simulink model "chenEx3p3p3_original"  (R2014a)
settings: Solver=ode45  StartTime=0.0  StopTime=10.0  RelTol=1e-3
values from neighbouring files (symbols this model uses):
  A = [-3.6         0       0   0 ... (first row only)    [chenEx3p3p3.m]    (also in chenEx3p3p3V3.m)
  B = [ 1 0 0 ... (first row only)    [chenEx3p3p3.m]    (also in chenEx3p3p3V3.m)
  C = [1    0   0   0 ... (first row only)    [chenEx3p3p3.m]    (also in chenEx3p3p3V3.m)
  C1 = C    [chenEx3p3p3.m]    (also in chenEx3p3p3V3.m)
  C2 = C    [chenEx3p3p3V3.m]
  C3 = C    [chenEx3p3p3V3.m]
  E = [1;20.758;0;0]    [chenEx3p3p3.m]    (also in chenEx3p3p3V3.m)
  F = A1-k1*C    [chenEx3p3p3.m]    (also in chenEx3p3p3V3.m)
  F1 = T1*A-k1*C    [chenEx3p3p3.m]    (also in chenEx3p3p3V3.m)
  H = E*inv((C*E)'*(C*E))*(C*E)'    [chenEx3p3p3.m]    (also in chenEx3p3p3V3.m)
  H1 = E1*inv((C*E1)'*(C*E1))*(C*E1)'    [chenEx3p3p3.m]    (also in chenEx3p3p3V3.m)
  H2 = E2*inv((C*E2)'*(C*E2))*(C*E2)'    [chenEx3p3p3.m]    (also in chenEx3p3p3V3.m)
  H3 = E3*inv((C*E3)'*(C*E3))*(C*E3)'    [chenEx3p3p3V3.m]
  k = k1 + F*H    [chenEx3p3p3.m]    (also in chenEx3p3p3V3.m)
  K1 = k1+F1*H1    [chenEx3p3p3.m]    (also in chenEx3p3p3V3.m)
  K2 = k2+F2*H2    [chenEx3p3p3.m]    (also in chenEx3p3p3V3.m)
  K3 = k3+F3*H3    [chenEx3p3p3V3.m]
  T = eye(4)-H*C    [chenEx3p3p3.m]    (also in chenEx3p3p3V3.m)
  T1 = eye(4) - H1*C    [chenEx3p3p3.m]    (also in chenEx3p3p3V3.m)
  T2 = eye(4) - H2*C    [chenEx3p3p3.m]    (also in chenEx3p3p3V3.m)
  T3 = eye(4) - H3*C    [chenEx3p3p3V3.m]
undefined symbols (not defined in the file or in its folder): C4, F4, H4, K, K4, T4
settings Model: Creator=sqn4594  LastModifiedBy=sqn4594
settings DataIOCC: SignalLoggingSaveFormat=ModelDataLogs
settings OptimizationCC: InitFltsAndDblsToZero=on
settings DebuggingCC: SaveWithParameterizedLinksMsg=none  UnderspecifiedInitializationDetection=Classic  SignalResolutionControl=TryResolveAllWithWarning  MultiTaskDSMMsg=warning  MultiTaskCondExecSysMsg=none
settings RTWCC: IncludeERTFirstTime=on
settings GRTTargetCC: TargetFcnLib=ansi_tfl_tmw.mat  CombineOutputUpdateFcns=off  GRTInterface=on

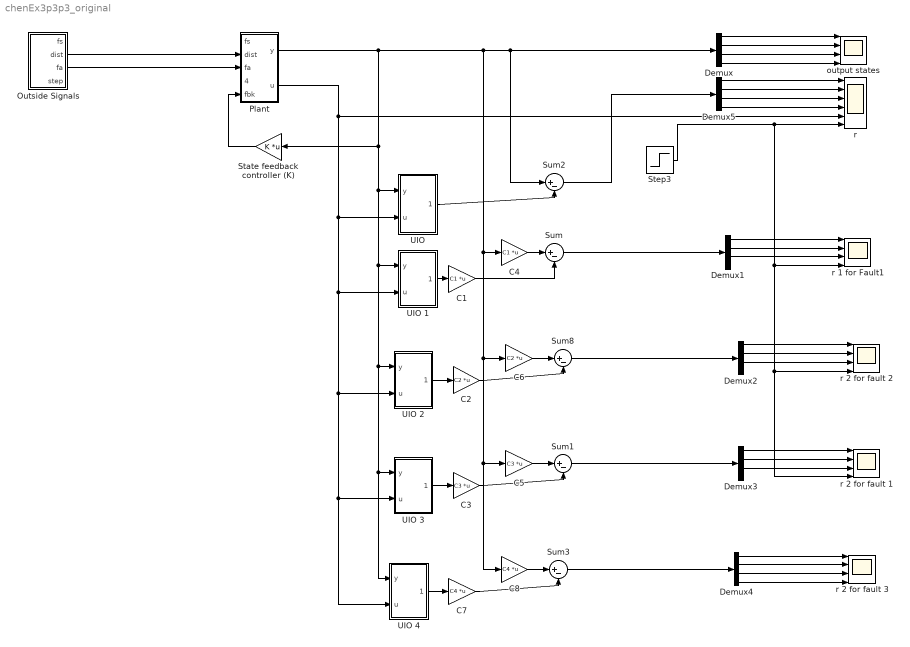
== system chenEx3p3p3_original ==
  C1 : Gain  Gain=C1  Multiplication=Matrix(K*u)
  C2 : Gain  Gain=C2  Multiplication=Matrix(K*u)
  C3 : Gain  Gain=C3  Multiplication=Matrix(K*u)
  C4 : Gain  Gain=C1  Multiplication=Matrix(K*u)
  C5 : Gain  Gain=C3  Multiplication=Matrix(K*u)
  C6 : Gain  Gain=C2  Multiplication=Matrix(K*u)
  C7 : Gain  Gain=C4  Multiplication=Matrix(K*u)
  C8 : Gain  Gain=C4  Multiplication=Matrix(K*u)
  Demux{,1..5} (6 alike) : Demux
  Outside Signals : Subsystem
  Plant : Subsystem
  State feedback controller (K) : Gain  Gain=K  Multiplication=Matrix(K*u)
  Step3 : Step  Time=7  SampleTime=0
  Sum{,1..3,8} (5 alike) : Sum  Inputs=|+-
  UIO : Subsystem
  UIO 1 : Subsystem
  UIO 2 : Subsystem
  UIO 3 : Subsystem
  UIO 4 : Subsystem
  output states : Scope  NumInputPorts=4
      settings: TimeRange=10  YMin=-5~-5~-5~-5  YMax=5~5~5~5
  r : Scope  NumInputPorts=6
      settings: YMin=-5~-5~-5~-5~-5~-5  YMax=5~5~5~5~5~5  SaveName=ScopeData5
  r 1 for Fault1 : Scope  NumInputPorts=4
      settings: YMin=-1e-020~-5~-5~-5  YMax=1e-020~5~5~5
  r 2 for fault 1 : Scope  NumInputPorts=4
      settings: YMin=-5~-5~-5~-5  YMax=5~5~5~5  SaveName=ScopeData3
  r 2 for fault 2 : Scope  NumInputPorts=4
      settings: YMin=-5~-5~-5~-5  YMax=5~5~5~5  SaveName=ScopeData2
  r 2 for fault 3 : Scope  NumInputPorts=4
      settings: YMin=-5~-5~-5~-5  YMax=5~5~5~5  SaveName=ScopeData4
  wires:
  Plant/1(y) -> State feedback controller (K)/1, UIO/1(y), UIO 1/1(y), UIO 2/1(y), UIO 3/1(y), UIO 4/1(y), Demux/1, Sum2/1, C4/1, C6/1, C5/1, C8/1
  Demux/2 -> output states/2
  Demux/3 -> output states/3
  Demux/4 -> output states/4
  Demux1/1 -> r 1 for Fault1/1
  State feedback controller (K)/1 -> Plant/5(fbk)
  Plant/2(u) -> UIO/2(u), UIO 1/2(u), UIO 2/2(u), UIO 3/2(u), UIO 4/2(u), r/5
  Step3/1 -> r/6, r 1 for Fault1/4, r 2 for fault 2/4, r 2 for fault 1/4
  UIO/1(ydot) -> Sum2/2
  Demux5/1 -> r/1
  Demux5/2 -> r/2
  Demux5/3 -> r/3
  Demux5/4 -> r/4
  Sum2/1 -> Demux5/1
  Demux/1 -> output states/1
  UIO 1/1(xdot) -> C1/1
  C1/1 -> Sum/2
  Demux1/2 -> r 1 for Fault1/2
  Demux1/3 -> r 1 for Fault1/3
  Sum/1 -> Demux1/1
  C4/1 -> Sum/1
  UIO 2/1(xdot) -> C2/1
  Demux2/1 -> r 2 for fault 2/1
  Demux2/2 -> r 2 for fault 2/2
  Demux2/3 -> r 2 for fault 2/3
  Sum8/1 -> Demux2/1
  C2/1 -> Sum8/2
  C6/1 -> Sum8/1
  UIO 3/1(xdot) -> C3/1
  Demux3/1 -> r 2 for fault 1/1
  Demux3/2 -> r 2 for fault 1/2
  Demux3/3 -> r 2 for fault 1/3
  Sum1/1 -> Demux3/1
  C3/1 -> Sum1/2
  C5/1 -> Sum1/1
  UIO 4/1(xdot) -> C7/1
  Demux4/1 -> r 2 for fault 3/1
  Demux4/2 -> r 2 for fault 3/2
  Demux4/3 -> r 2 for fault 3/3
  Sum3/1 -> Demux4/1
  C7/1 -> Sum3/2
  Demux4/4 -> r 2 for fault 3/4
  C8/1 -> Sum3/1
  Outside Signals/3(fa) -> Plant/3(fa)
  Outside Signals/2(dist) -> Plant/2(dist)

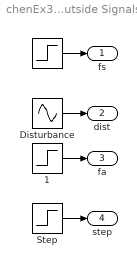
== system chenEx3p3p3_original/Outside Signals ==
  "  " : Step  Time=7  SampleTime=0
  "  1" : Step  Time=7  SampleTime=0
  Disturbance : Sin  Frequency=100  SampleTime=0
  Step : Step  Time=0  SampleTime=0
  fs : Outport
  dist : Outport  Port=2
  fa : Outport  Port=3
  "step " : Outport  Port=4
  wires:
  "  "/1 -> fs/1
  Disturbance/1 -> dist/1
  "  1"/1 -> fa/1
  Step/1 -> "step "/1

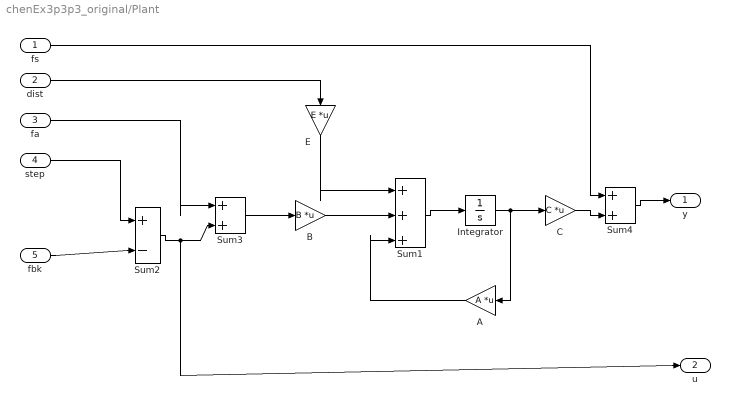
== system chenEx3p3p3_original/Plant ==
  fs : Inport
  dist : Inport  Port=2
  fa : Inport  Port=3
  step : Inport  Port=4
  fbk : Inport  Port=5
  A : Gain  Gain=A  Multiplication=Matrix(K*u)
  B : Gain  Gain=B  Multiplication=Matrix(K*u)
  C : Gain  Gain=C  Multiplication=Matrix(K*u)
  E : Gain  Gain=E  Multiplication=Matrix(K*u)
  Integrator : Integrator  InitialCondition=[.01;0;.011;.011]
  Sum1 : Sum  Inputs=|+++
  Sum2 : Sum  Inputs=|+-
  Sum3 : Sum  Inputs=|++
  Sum4 : Sum  Inputs=|++
  y : Outport
  u : Outport  Port=2
  wires:
  Sum1/1 -> Integrator/1
  step/1 -> Sum2/1
  fbk/1 -> Sum2/2
  Integrator/1 -> C/1, A/1
  Sum2/1 -> Sum3/2, u/1
  B/1 -> Sum1/2
  Sum3/1 -> B/1
  C/1 -> Sum4/2
  A/1 -> Sum1/3
  E/1 -> Sum1/1
  Sum4/1 -> y/1
  fa/1 -> Sum3/1
  dist/1 -> E/1
  fs/1 -> Sum4/1

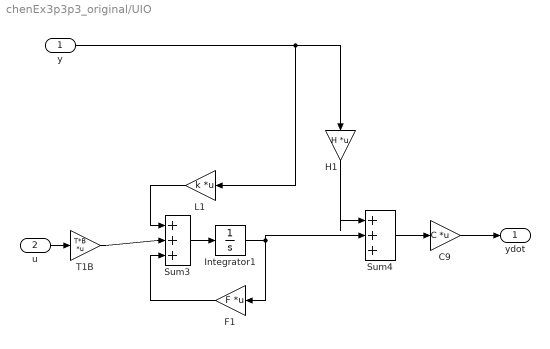
== system chenEx3p3p3_original/UIO ==
  y : Inport
  u : Inport  Port=2
  C9 : Gain  Gain=C  Multiplication=Matrix(K*u)
  F1 : Gain  Gain=F  Multiplication=Matrix(K*u)
  H1 : Gain  Gain=H  Multiplication=Matrix(K*u)
  Integrator1 : Integrator
  L1 : Gain  Gain=k  Multiplication=Matrix(K*u)
  Sum3 : Sum  Inputs=|+++
  Sum4 : Sum  Inputs=|+++
  T1B : Gain  Gain=T*B  Multiplication=Matrix(K*u)
  ydot : Outport
  wires:
  Sum3/1 -> Integrator1/1
  Integrator1/1 -> F1/1, Sum4/2
  F1/1 -> Sum3/3
  L1/1 -> Sum3/1
  T1B/1 -> Sum3/2
  H1/1 -> Sum4/1
  Sum4/1 -> C9/1
  y/1 -> L1/1, H1/1
  u/1 -> T1B/1
  C9/1 -> ydot/1

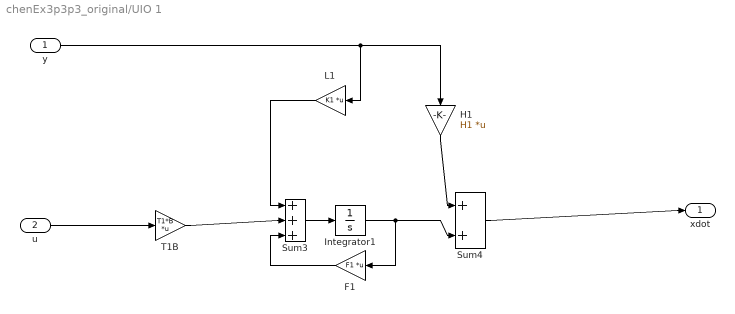
== system chenEx3p3p3_original/UIO 1 ==
  y : Inport
  u : Inport  Port=2
  F1 : Gain  Gain=F1  Multiplication=Matrix(K*u)
  H1 : Gain  Gain=H1  Multiplication=Matrix(K*u)
  Integrator1 : Integrator
  L1 : Gain  Gain=K1  Multiplication=Matrix(K*u)
  Sum3 : Sum  Inputs=|+++
  Sum4 : Sum  Inputs=|++
  T1B : Gain  Gain=T1*B  Multiplication=Matrix(K*u)
  xdot : Outport
  wires:
  Sum3/1 -> Integrator1/1
  Integrator1/1 -> Sum4/2, F1/1
  F1/1 -> Sum3/3
  L1/1 -> Sum3/1
  T1B/1 -> Sum3/2
  H1/1 -> Sum4/1
  u/1 -> T1B/1
  Sum4/1 -> xdot/1
  y/1 -> H1/1, L1/1

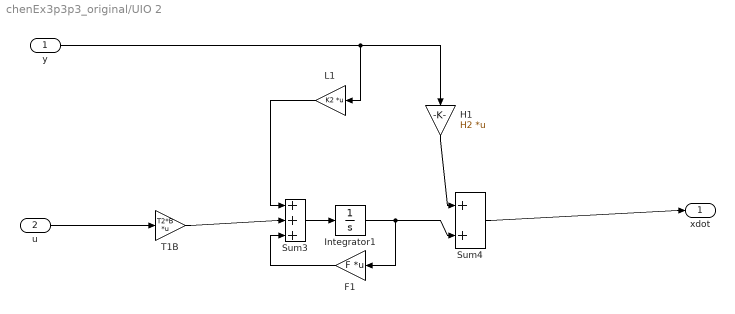
== system chenEx3p3p3_original/UIO 2 ==
  y : Inport
  u : Inport  Port=2
  F1 : Gain  Gain=F  Multiplication=Matrix(K*u)
  H1 : Gain  Gain=H2  Multiplication=Matrix(K*u)
  Integrator1 : Integrator
  L1 : Gain  Gain=K2  Multiplication=Matrix(K*u)
  Sum3 : Sum  Inputs=|+++
  Sum4 : Sum  Inputs=|++
  T1B : Gain  Gain=T2*B  Multiplication=Matrix(K*u)
  xdot : Outport
  wires:
  Sum3/1 -> Integrator1/1
  Integrator1/1 -> Sum4/2, F1/1
  F1/1 -> Sum3/3
  L1/1 -> Sum3/1
  T1B/1 -> Sum3/2
  H1/1 -> Sum4/1
  u/1 -> T1B/1
  Sum4/1 -> xdot/1
  y/1 -> H1/1, L1/1

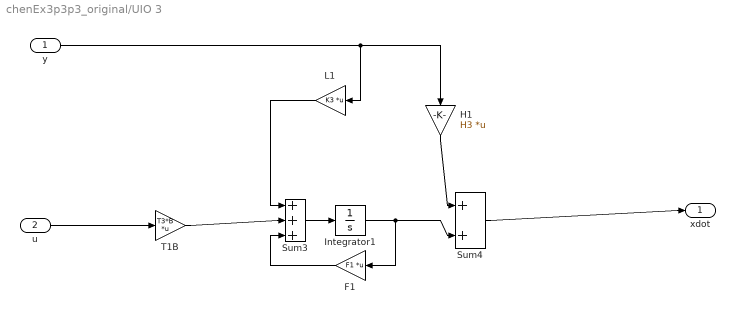
== system chenEx3p3p3_original/UIO 3 ==
  y : Inport
  u : Inport  Port=2
  F1 : Gain  Gain=F1  Multiplication=Matrix(K*u)
  H1 : Gain  Gain=H3  Multiplication=Matrix(K*u)
  Integrator1 : Integrator
  L1 : Gain  Gain=K3  Multiplication=Matrix(K*u)
  Sum3 : Sum  Inputs=|+++
  Sum4 : Sum  Inputs=|++
  T1B : Gain  Gain=T3*B  Multiplication=Matrix(K*u)
  xdot : Outport
  wires:
  Sum3/1 -> Integrator1/1
  Integrator1/1 -> Sum4/2, F1/1
  F1/1 -> Sum3/3
  L1/1 -> Sum3/1
  T1B/1 -> Sum3/2
  H1/1 -> Sum4/1
  u/1 -> T1B/1
  Sum4/1 -> xdot/1
  y/1 -> H1/1, L1/1

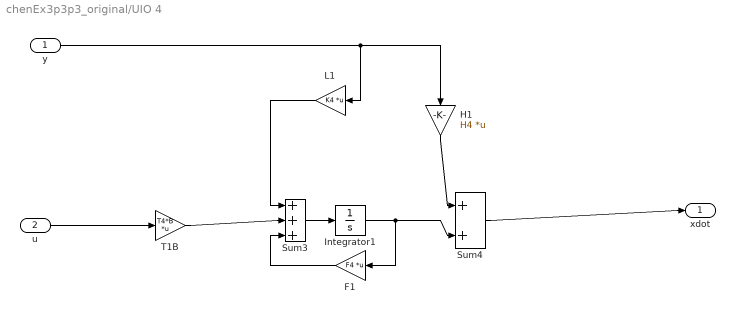
== system chenEx3p3p3_original/UIO 4 ==
  y : Inport
  u : Inport  Port=2
  F1 : Gain  Gain=F4  Multiplication=Matrix(K*u)
  H1 : Gain  Gain=H4  Multiplication=Matrix(K*u)
  Integrator1 : Integrator
  L1 : Gain  Gain=K4  Multiplication=Matrix(K*u)
  Sum3 : Sum  Inputs=|+++
  Sum4 : Sum  Inputs=|++
  T1B : Gain  Gain=T4*B  Multiplication=Matrix(K*u)
  xdot : Outport
  wires:
  Sum3/1 -> Integrator1/1
  Integrator1/1 -> Sum4/2, F1/1
  F1/1 -> Sum3/3
  L1/1 -> Sum3/1
  T1B/1 -> Sum3/2
  H1/1 -> Sum4/1
  u/1 -> T1B/1
  Sum4/1 -> xdot/1
  y/1 -> H1/1, L1/1
